simulink model "AmplitudeModulationSimulink"  (R2021a)
settings: Solver=VariableStepAuto  StartTime=0.0  StopTime=10.0  RelTol=1e-3
settings Model: Creator=Arif  LastModifiedBy=Arif

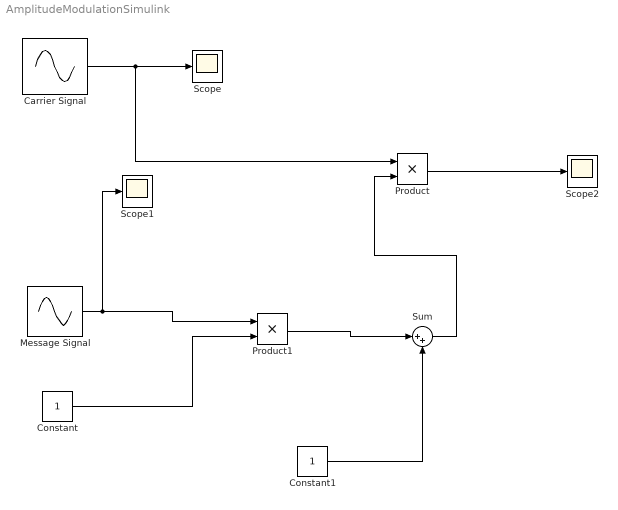
== system AmplitudeModulationSimulink ==
  Carrier Signal : Sin  Frequency=2*pi*25  SampleTime=0.0005
  Constant : Constant
  Constant1 : Constant
  Message Signal : Sin  Frequency=2*pi  SampleTime=0.0005
  Product : Product
  Product1 : Product
  Scope : Scope
  Scope1 : Scope
  Scope2 : Scope
  Sum : Sum  Inputs=|++
  wires:
  Carrier Signal/1 -> Product/1, Scope/1
  Message Signal/1 -> Product1/1, Scope1/1
  Constant/1 -> Product1/2
  Constant1/1 -> Sum/2
  Product1/1 -> Sum/1
  Sum/1 -> Product/2
  Product/1 -> Scope2/1
